simulink model "compensation"  (R2019a)
settings: Solver=FixedStepAuto  StartTime=0.0  StopTime=Ncyc  RelTol=1e-3  EnableMultiTasking=on
values from neighbouring files (symbols this model uses):
  kc = (Tc/(k*Kp_id))*p1*p2    [Compensator.m]
  Kp_d = 31    [Compensator.m]
  r = 60    [Compensator.m]
  r_cyc = 4000*ts    (= 200)    [Compensator.m]
  T = 0.2024    [Compensator.m]
  Tc = -1/(p1+p2)    [Compensator.m]
  ts = 1/freq    (= 0.05)    [Compensator.m]
libraries: arduinolib x3
settings Model: ExtModeTrigDuration=2  Creator=xde12  LastModifiedBy=xde12
settings DataIOCC: ReturnWorkspaceOutputs=off
settings OptimizationCC: EnhancedBackFolding=on  PassReuseOutputArgsThreshold=0  MaxStackSize=64  OptimizeBlockOrder=speed  DifferentSizesBufferReuse=on  OptimizationCustomize=off
settings DebuggingCC: ParameterTunabilityLossMsg=error  PregeneratedLibrarySubsystemCodeDiagnostic=none  ArithmeticOperatorsInVariantConditions=warning
settings HardwareCC: ProdBitPerInt=16  ProdBitPerPointer=16  ProdBitPerSizeT=16  ProdBitPerPtrDiffT=16  ProdLargestAtomicFloat=None  ProdWordSize=8  ProdHWDeviceType=Atmel->AVR  UseEmbeddedCoderFeatures=off  UseSimulinkCoderFeatures=off
settings SFSimCC: SimUseLocalCustomCode=off  MATLABDynamicMemAlloc=off
settings RTWCC: SystemTargetFile=ert.tlc  HardwareBoard=Arduino Uno  TLCOptions=-aInlineSetEventsForThisBaseRateFcn=TLC_FALSE -aSuppressMultiTaskScheduler=TLC_FALSE -aRateBasedStepFcn=1  TemplateMakefile=ert_default_tmf  GenerateReport=on  RTWUseLocalCustomCode=off  Toolchain=Arduino AVR  BuildConfiguration=Faster Runs  LaunchReport=on
settings CodeAppCC: ForceParamTrailComments=on  OperatorAnnotations=on
settings ERTTargetCC: ERTCustomFileBanners=off  SupportContinuousTime=on  SupportNonInlinedSFcns=on  RemoveResetFunc=off  SupportVariableSizeSignals=on  ModelStepFunctionPrototypeControlCompliant=off

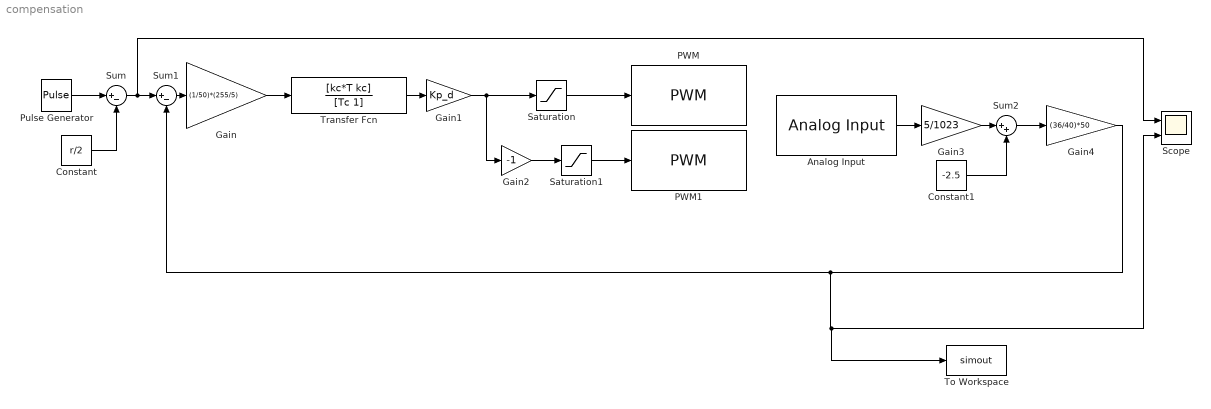
== system compensation ==
  Analog Input : arduinolib/Analog Input  pinNumber=0  ReadResultsOnly=off  ConversionTriggerSource=Software  ExternalTriggerType=uint32(0)  OutputDataType=uint16  EnableConversionCompleteNotify=off  EnableOuputStatus=off  SampleTime=ts  blockPlatform=arduino
  Constant : Constant  Value=r/2  SampleTime=ts
  Constant1 : Constant  Value=-2.5  SampleTime=ts
  Gain : Gain  Gain=(1/50)*(255/5)
  Gain1 : Gain  Gain=Kp_d
  Gain2 : Gain  Gain=-1
  Gain3 : Gain  Gain=5/1023
  Gain4 : Gain  Gain=(36/40)*50
  PWM : arduinolib/PWM  pinNumber=3  EnableInputFrequency=off  InitialFrequency=2000  InitialDutyCycle=0  NotificationType=None  blockPlatform=arduino
  PWM1 : arduinolib/PWM  pinNumber=5  EnableInputFrequency=off  InitialFrequency=2000  InitialDutyCycle=0  NotificationType=None  blockPlatform=arduino
  Pulse Generator : DiscretePulseGenerator  Amplitude=r  Period=r_cyc  PulseWidth=r_cyc/2  SampleTime=ts
  Saturation : Saturate  UpperLimit=255  LowerLimit=0
  Saturation1 : Saturate  UpperLimit=255  LowerLimit=0
  Scope : Scope  NumInputPorts=2
  Sum : Sum  Inputs=|+-
  Sum1 : Sum  Inputs=|+-
  Sum2 : Sum  Inputs=|++
  To Workspace : ToWorkspace  VariableName=simout  SampleTime=-1
      settings: Save2DSignal=2-D array (concatenate along first dimension)
  Transfer Fcn : TransferFcn  Numerator=[kc*T kc]  Denominator=[Tc 1]
  wires:
  Analog Input/1 -> Gain3/1
  Pulse Generator/1 -> Sum/1
  Sum/1 -> Scope/1, Sum1/1
  Sum1/1 -> Gain/1
  Gain1/1 -> Gain2/1, Saturation/1
  Constant/1 -> Sum/2
  Gain2/1 -> Saturation1/1
  Saturation1/1 -> PWM1/1
  Saturation/1 -> PWM/1
  Sum2/1 -> Gain4/1
  Gain3/1 -> Sum2/1
  Gain4/1 -> To Workspace/1, Scope/2, Sum1/2
  Constant1/1 -> Sum2/2
  Gain/1 -> Transfer Fcn/1
  Transfer Fcn/1 -> Gain1/1
